simulink model "ChirpTest_ParameterEstimation"  (R2019b)
settings: Solver=VariableStepAuto  StartTime=0.0  StopTime=chirp_t_end  MaxStep=1/(PWM_Resolution*PWM_Frequency)  RelTol=1e-3
PreLoadFcn:
  | modelDir = fileparts(get_param(bdroot, 'FileName'));
  | addpath(fullfile(modelDir,'../Parameters'));
  | addpath(fullfile(modelDir,'subsystems'));
  | addpath(fullfile(modelDir,'../DesignExploration/functions')); % for PWM_Generator
  | 
  | Parameters_Model
  | Parameters_Simulation
  | Parameters_Estimators
  | Parameters_Test_Chirp
InitFcn:
  | Parameters_Model
  | Parameters_Simulation
  | Parameters_Test_Chirp
  | Parameters_Estimators
undefined symbols (not defined in the file): chirp_duty_cycle, chirp_freq_end, chirp_freq_start, chirp_t_end, EnableNoise, sensor_sigma2_current_sense
libraries: simulink x8
settings Model: Creator=Thomas  LastModifiedBy=thomas.jespersen
settings DataIOCC: ReturnWorkspaceOutputs=off
settings DebuggingCC: ArithmeticOperatorsInVariantConditions=warning
settings SFSimCC: SimUseLocalCustomCode=off  CustomCodeUndefinedFunction=UseInterfaceOnly
settings RTWCC: RTWUseLocalCustomCode=off

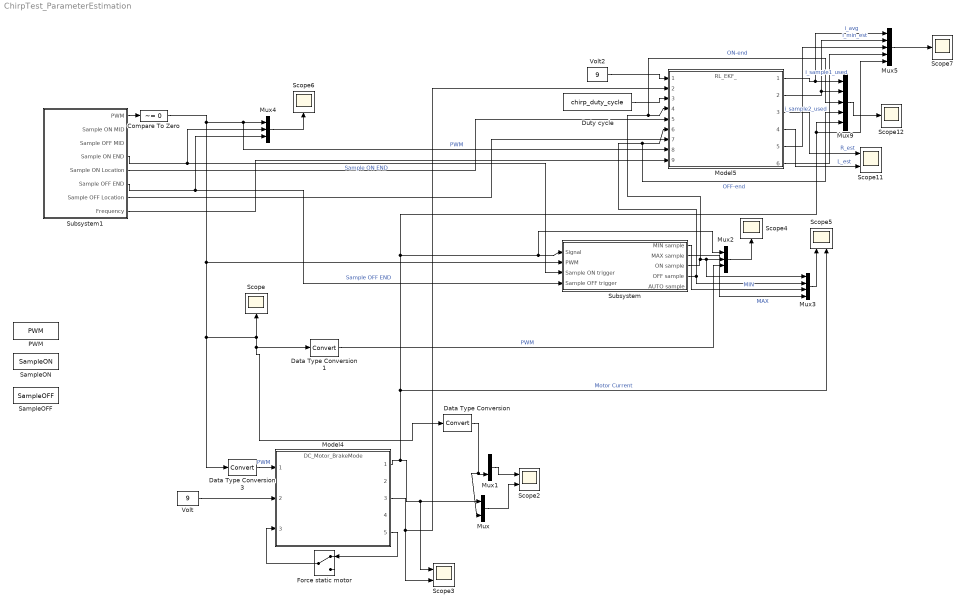
== system ChirpTest_ParameterEstimation ==
  Compare To Zero : simulink/Logic and Bit Operations/Compare To Zero  relop=~=  OutDataTypeStr=boolean
  Data Type Conversion : DataTypeConversion  RndMeth=Round
  Data Type Conversion1 : DataTypeConversion  RndMeth=Round
  Data Type Conversion3 : DataTypeConversion  RndMeth=Round
  Duty cycle : Constant  Value=chirp_duty_cycle
  Force static motor : ManualSwitch
  Model4 : ModelReference  ModelNameDialog=DC_Motor_BrakeMode  SimulationMode=Normal  ModelReferenceVersion=1.43
  Model5 : ModelReference  ModelNameDialog=RL_EKF_  SimulationMode=Normal  ModelReferenceVersion=1.70
  Mux : Mux  Inputs=2
  Mux1 : Mux  Inputs=2
  Mux2 : Mux  Inputs=3
  Mux3 : Mux
  Mux4 : Mux  Inputs=3
  Mux5 : Mux  Inputs=5
  Mux9 : Mux  Inputs=5
  PWM : FromWorkspace  VariableName=PWM  SampleTime=0  Interpolate=off  OutputAfterFinalValue=Holding final value
  SampleOFF : FromWorkspace  VariableName=SampleOFF  SampleTime=0  Interpolate=off  OutputAfterFinalValue=Holding final value
  SampleON : FromWorkspace  VariableName=SampleON  SampleTime=0  Interpolate=off  OutputAfterFinalValue=Holding final value
  Scope{,4,6..7,12} (5 alike) : Scope
  Scope{2..3,5,11} (4 alike) : Scope  NumInputPorts=2
  Subsystem : Subsystem
  Subsystem1 : Subsystem
  Volt : Constant  Value=9
  Volt2 : Constant  Value=9
  wires:
  Volt/1 -> Model4/2
  Mux/1 -> Scope2/2
  Mux1/1 -> Scope2/1
  Data Type Conversion/1 -> Mux/2, Mux1/2
  Model4/3 -> Model5/2, Scope3/2
  Mux2/1 -> Scope4/1
  Subsystem/3(ON sample) -> Mux9/3, Model5/4, Mux3/1, Mux2/2  "ON-end"
  Mux3/1 -> Scope5/1
  Subsystem/4(OFF sample) -> Mux3/2, Mux9/4, Model5/6  "OFF-end"
  Subsystem/1(MIN sample) -> Mux3/3  "MIN"
  Subsystem/2(MAX sample) -> Mux3/4  "MAX"
  Model4/5 -> Force static motor/1
  Force static motor/1 -> Model4/3
  Data Type Conversion1/1 -> Mux2/3  "PWM"
  Mux4/1 -> Scope6/1
  Subsystem1/4(Sample ON END) -> Mux4/2, Subsystem/3(Sample ON trigger)  "Sample ON END"
  Subsystem1/6(Sample OFF END) -> Mux4/3, Subsystem/4(Sample OFF trigger)  "Sample OFF END"
  Volt2/1 -> Model5/1
  Duty cycle/1 -> Model5/3
  Subsystem1/5(Sample ON Location) -> Model5/5
  Subsystem1/7(Sample OFF Location) -> Model5/7
  Mux9/1 -> Scope12/1
  Model5/1 -> Mux5/1, Mux9/1  "i_avg"
  Model5/2 -> Mux5/2, Mux9/2  "i_min_est"
  Model5/3 -> Scope11/1  "R_est"
  Model5/4 -> Scope11/2  "L_est"
  Mux5/1 -> Scope7/1
  Model5/5 -> Mux5/3  "i_sample1_used"
  Model5/6 -> Mux5/4  "i_sample2_used"
  Model4/1 -> Scope5/2, Mux5/5, Mux9/5, Mux2/1, Subsystem/1(Signal), Scope3/1, Mux/1  "Motor Current"
  Subsystem1/8(Frequency) -> Model5/9
  Subsystem1/1(PWM) -> Compare To Zero/1
  Data Type Conversion3/1 -> Model4/1  "PWM"
  Compare To Zero/1 -> Data Type Conversion3/1, Data Type Conversion1/1, Data Type Conversion/1, Scope/1, Subsystem/2(PWM), Model5/8, Mux4/1  "PWM"

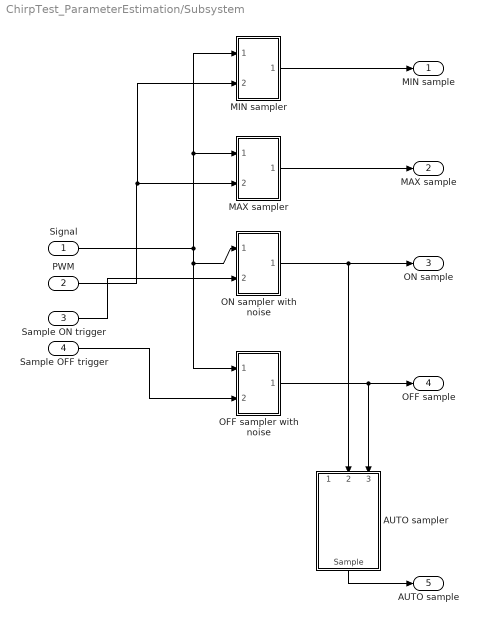
== system ChirpTest_ParameterEstimation/Subsystem ==
  Signal : Inport
  PWM : Inport  Port=2
  Sample ON trigger : Inport  Port=3
  Sample OFF trigger : Inport  Port=4
  AUTO sampler : Subsystem
  MAX sampler : Subsystem
  MIN sampler : Subsystem
  OFF sampler with noise : Subsystem
  ON sampler with noise : Subsystem
  MIN sample : Outport  VectorParamsAs1DForOutWhenUnconnected=off
  MAX sample : Outport  Port=2  VectorParamsAs1DForOutWhenUnconnected=off
  ON sample : Outport  Port=3  VectorParamsAs1DForOutWhenUnconnected=off
  OFF sample : Outport  Port=4  VectorParamsAs1DForOutWhenUnconnected=off
  AUTO sample : Outport  Port=5  VectorParamsAs1DForOutWhenUnconnected=off
  wires:
  Signal/1 -> OFF sampler with noise/1(Signal), ON sampler with noise/1(Signal), MAX sampler/1(Signal), MIN sampler/1(Signal)
  ON sampler with noise/1(Sample) -> AUTO sampler/2(ON sample), ON sample/1
  OFF sampler with noise/1(Sample) -> AUTO sampler/3(OFF sample), OFF sample/1
  AUTO sampler/1(Sample) -> AUTO sample/1
  MAX sampler/1(Sample) -> MAX sample/1
  MIN sampler/1(Sample) -> MIN sample/1
  PWM/1 -> MIN sampler/2(PWM), MAX sampler/2(PWM)
  Sample OFF trigger/1 -> OFF sampler with noise/2(Trigger)
  Sample ON trigger/1 -> ON sampler with noise/2(Trigger)

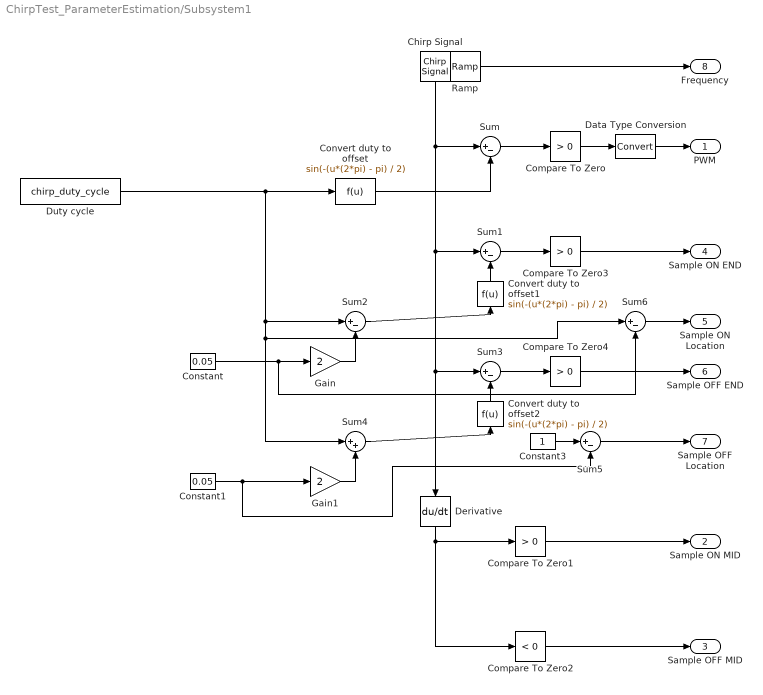
== system ChirpTest_ParameterEstimation/Subsystem1 ==
  Chirp Signal : simulink/Sources/Chirp Signal  f1=chirp_freq_end  T=chirp_t_end  f2=chirp_freq_start
  Compare To Zero : simulink/Logic and Bit Operations/Compare To Zero  relop=>  OutDataTypeStr=boolean
  Compare To Zero1 : simulink/Logic and Bit Operations/Compare To Zero  relop=>  OutDataTypeStr=boolean  ZeroCross=off
  Compare To Zero2 : simulink/Logic and Bit Operations/Compare To Zero  relop=<  OutDataTypeStr=boolean  ZeroCross=off
  Compare To Zero3 : simulink/Logic and Bit Operations/Compare To Zero  relop=>  OutDataTypeStr=boolean
  Compare To Zero4 : simulink/Logic and Bit Operations/Compare To Zero  relop=>  OutDataTypeStr=boolean
  Constant : Constant  Value=0.05
  Constant1 : Constant  Value=0.05
  Constant3 : Constant
  Convert duty to offset : Fcn  Expr=sin(-(u*(2*pi) - pi) / 2)
  Convert duty to offset1 : Fcn  Expr=sin(-(u*(2*pi) - pi) / 2)
  Convert duty to offset2 : Fcn  Expr=sin(-(u*(2*pi) - pi) / 2)
  Data Type Conversion : DataTypeConversion  RndMeth=Round
  Derivative : Derivative
  Duty cycle : Constant  Value=chirp_duty_cycle
  Gain : Gain  Gain=2
  Gain1 : Gain  Gain=2
  Ramp : simulink/Sources/Ramp  slope=(chirp_freq_start-chirp_freq_end)/chirp_t_end  start=0  InitialOutput=chirp_freq_end
  Sum{,1..3,5..6} (6 alike) : Sum  Inputs=|+-
  Sum4 : Sum  Inputs=|++
  PWM : Outport  OutDataTypeStr=int8  VectorParamsAs1DForOutWhenUnconnected=off
  Sample ON MID : Outport  Port=2  VectorParamsAs1DForOutWhenUnconnected=off
  Sample OFF MID : Outport  Port=3  VectorParamsAs1DForOutWhenUnconnected=off
  Sample ON END : Outport  Port=4  VectorParamsAs1DForOutWhenUnconnected=off
  Sample ON Location : Outport  Port=5  VectorParamsAs1DForOutWhenUnconnected=off
  Sample OFF END : Outport  Port=6  VectorParamsAs1DForOutWhenUnconnected=off
  Sample OFF Location : Outport  Port=7  VectorParamsAs1DForOutWhenUnconnected=off
  Frequency : Outport  Port=8  VectorParamsAs1DForOutWhenUnconnected=off
  wires:
  Sum/1 -> Compare To Zero/1
  Convert duty to offset/1 -> Sum/2
  Compare To Zero/1 -> Data Type Conversion/1
  Compare To Zero1/1 -> Sample ON MID/1
  Compare To Zero2/1 -> Sample OFF MID/1
  Derivative/1 -> Compare To Zero2/1, Compare To Zero1/1
  Sum2/1 -> Convert duty to offset1/1
  Compare To Zero3/1 -> Sample ON END/1
  Chirp Signal/1 -> Sum1/1, Sum3/1, Derivative/1, Sum/1
  Sum1/1 -> Compare To Zero3/1
  Convert duty to offset1/1 -> Sum1/2
  Convert duty to offset2/1 -> Sum3/2
  Sum4/1 -> Convert duty to offset2/1
  Sum3/1 -> Compare To Zero4/1
  Compare To Zero4/1 -> Sample OFF END/1
  Constant1/1 -> Sum5/2, Gain1/1
  Sum5/1 -> Sample OFF Location/1
  Constant3/1 -> Sum5/1
  Constant/1 -> Sum6/2, Gain/1
  Duty cycle/1 -> Sum6/1, Sum4/1, Sum2/1, Convert duty to offset/1
  Gain/1 -> Sum2/2
  Sum6/1 -> Sample ON Location/1
  Gain1/1 -> Sum4/2
  Ramp/1 -> Frequency/1
  Data Type Conversion/1 -> PWM/1

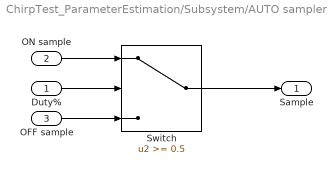
== system ChirpTest_ParameterEstimation/Subsystem/AUTO sampler ==
  Duty% : Inport  OutDataTypeStr=double
  ON sample : Inport  Port=2
  OFF sample : Inport  Port=3
  Switch : Switch  Threshold=0.5
  Sample : Outport  VectorParamsAs1DForOutWhenUnconnected=off
  wires:
  Duty%/1 -> Switch/2
  ON sample/1 -> Switch/1
  OFF sample/1 -> Switch/3
  Switch/1 -> Sample/1

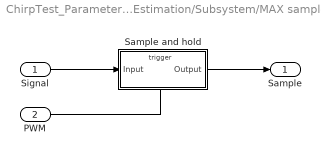
== system ChirpTest_ParameterEstimation/Subsystem/MAX sampler ==
  Signal : Inport
  PWM : Inport  Port=2
  Sample and hold : Subsystem
  Sample : Outport  VectorParamsAs1DForOutWhenUnconnected=off
  wires:
  Signal/1 -> Sample and hold/1(Input)
  Sample and hold/1(Output) -> Sample/1
  PWM/1 -> Sample and hold/Trigger

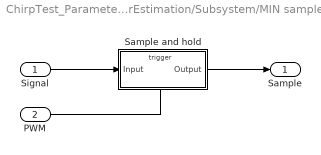
== system ChirpTest_ParameterEstimation/Subsystem/MIN sampler ==
  Signal : Inport
  PWM : Inport  Port=2
  Sample and hold : Subsystem
  Sample : Outport  VectorParamsAs1DForOutWhenUnconnected=off
  wires:
  Signal/1 -> Sample and hold/1(Input)
  Sample and hold/1(Output) -> Sample/1
  PWM/1 -> Sample and hold/Trigger

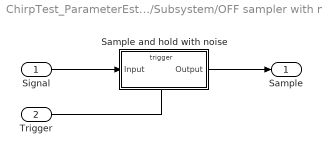
== system ChirpTest_ParameterEstimation/Subsystem/OFF sampler with noise ==
  Signal : Inport
  Trigger : Inport  Port=2
  Sample and hold with noise : Subsystem
  Sample : Outport  VectorParamsAs1DForOutWhenUnconnected=off
  wires:
  Signal/1 -> Sample and hold with noise/1(Input)
  Sample and hold with noise/1(Output) -> Sample/1
  Trigger/1 -> Sample and hold with noise/Trigger

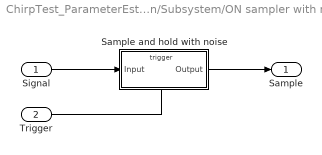
== system ChirpTest_ParameterEstimation/Subsystem/ON sampler with noise ==
  Signal : Inport
  Trigger : Inport  Port=2
  Sample and hold with noise : Subsystem
  Sample : Outport  VectorParamsAs1DForOutWhenUnconnected=off
  wires:
  Signal/1 -> Sample and hold with noise/1(Input)
  Sample and hold with noise/1(Output) -> Sample/1
  Trigger/1 -> Sample and hold with noise/Trigger

== system ChirpTest_ParameterEstimation/Subsystem/MAX sampler/Sample and hold ==
  Input : Inport
  Trigger : TriggerPort  TriggerType=falling  VariantControl=Variant  PortDimensions=1
  Output : Outport  VectorParamsAs1DForOutWhenUnconnected=off
  wires:
  Input/1 -> Output/1

== system ChirpTest_ParameterEstimation/Subsystem/MIN sampler/Sample and hold ==
  Input : Inport
  Trigger : TriggerPort  VariantControl=Variant  PortDimensions=1
  Output : Outport  VectorParamsAs1DForOutWhenUnconnected=off
  wires:
  Input/1 -> Output/1

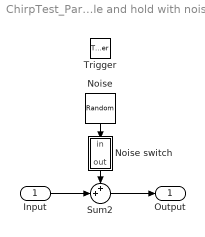
== system ChirpTest_ParameterEstimation/Subsystem/OFF sampler with noise/Sample and hold with noise ==
  Input : Inport
  Trigger : TriggerPort  VariantControl=Variant  PortDimensions=1
  Noise : RandomNumber  Variance=sensor_sigma2_current_sense  Seed=32
  Noise switch : Subsystem
  Sum2 : Sum  Inputs=++|
  Output : Outport  VectorParamsAs1DForOutWhenUnconnected=off
  wires:
  Noise/1 -> Noise switch/1(in)
  Noise switch/1(out) -> Sum2/1
  Input/1 -> Sum2/2
  Sum2/1 -> Output/1

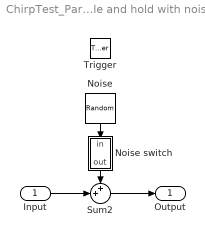
== system ChirpTest_ParameterEstimation/Subsystem/ON sampler with noise/Sample and hold with noise ==
  Input : Inport
  Trigger : TriggerPort  TriggerType=falling  VariantControl=Variant  PortDimensions=1
  Noise : RandomNumber  Variance=sensor_sigma2_current_sense  Seed=55
  Noise switch : Subsystem
  Sum2 : Sum  Inputs=++|
  Output : Outport  VectorParamsAs1DForOutWhenUnconnected=off
  wires:
  Noise/1 -> Noise switch/1(in)
  Noise switch/1(out) -> Sum2/1
  Input/1 -> Sum2/2
  Sum2/1 -> Output/1

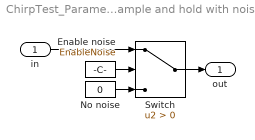
== system ChirpTest_ParameterEstimation/Subsystem/OFF sampler with noise/Sample and hold with noise/Noise switch ==
  in : Inport
  Enable noise : Constant  Value=EnableNoise
  No noise : Constant  Value=0
  Switch : Switch  Criteria=u2 > Threshold
  out : Outport  VectorParamsAs1DForOutWhenUnconnected=off
  wires:
  No noise/1 -> Switch/3
  Switch/1 -> out/1
  Enable noise/1 -> Switch/2
  in/1 -> Switch/1

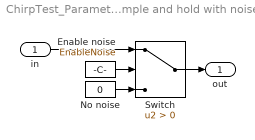
== system ChirpTest_ParameterEstimation/Subsystem/ON sampler with noise/Sample and hold with noise/Noise switch ==
  in : Inport
  Enable noise : Constant  Value=EnableNoise
  No noise : Constant  Value=0
  Switch : Switch  Criteria=u2 > Threshold
  out : Outport  VectorParamsAs1DForOutWhenUnconnected=off
  wires:
  No noise/1 -> Switch/3
  Switch/1 -> out/1
  Enable noise/1 -> Switch/2
  in/1 -> Switch/1
